simulink model "model_4"  (R2020a)
settings: Solver=VariableStepAuto  StartTime=0.0  StopTime=10.0  RelTol=1e-3
settings Model: Creator=Notnik_kg  LastModifiedBy=Notnik_kg

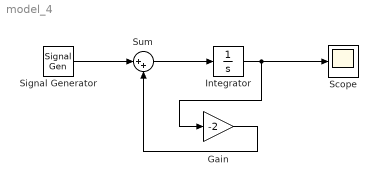
== system model_4 ==
  Gain : Gain  Gain=-2
  Integrator : Integrator
  Scope : Scope
  Signal Generator : SignalGenerator  WaveForm=square  Units=rad/sec
  Sum : Sum  Inputs=|++
  wires:
  Signal Generator/1 -> Sum/1
  Sum/1 -> Integrator/1
  Integrator/1 -> Scope/1, Gain/1
  Gain/1 -> Sum/2
